simulink library "Control_System_Library"  (Simulink 8.0)
settings: Solver=ode45  StartTime=0.0  StopTime=10.0  RelTol=1e-3
values from neighbouring files (symbols this model uses):
  B_bias = [0 0 0]    [Initialize_UKF_Function.m]
  B_Init_Inertial = wrldmagm(Alt, Lat, Long, 2013)*1E-9    [Initialize_UKF_Function.m]
  I_c = [3.4 3.4 1.9]    [Initialize_UKF_Function.m]    (also in UKF_quaternion_withBias.m)
  NED_Init = dcmecef2ned(Lat, Long)*ECEF_Init    [Initialize_UKF_Function.m]
  q_i_s0 = init_attitude    [Initialize_UKF_Function.m]
  q_s_c = [1 0 0 0]    [Initialize_UKF_Function.m]    (also in Satellite2Controller_Conversion.m = dcm2quat(R); UKF_quaternion_withBias.m = [1; 0; 0; 0])
  Time_Start = 0    [Initialize_UKF_Function.m]
  Ts = .1    (= 0.1)    [Initialize_UKF_Function.m]
  w_bias = 0*[0.5 0.2 0.15]    [Initialize_UKF_Function.m]    (also in UKF_quaternion_withBias.m = zeros(3,1))
  w_init_s = [rand_w_x rand_w_y rand_w_z]    [Initialize_UKF_Function.m]
undefined symbols (not defined in the file or in its folder): aeroassertmsg, c, cd, DiscIntNeverNeededParam, dyear, Earth, epoch, fm, fn, k, maxdef, Newton, Raphson, sgp4, snorm, WGS84
libraries: commnoisgen2 x6, aerolibconvert2 x4, simulink x3, aerolibutil x2, aerolibtransform2 x2, dspmtrx3 x1, aerolibgravitysys x1
(part 3 of 3)

== matlab function Dynamic Model/Aerodynamic and Atmospheric Disturbance Torque Model/MATLAB Function1 ==
  data: Solar_Torque output double
function Solar_Torque = Solar_Drag_Torque()
% Solar_Drag_Torque
% Author: Brandon Jackson
% Contact: bajackso@mtu.edu
% Date: 26 June 2013
%
% Description: This function performs an analysis on the solar density
% above a fixed location of the Earth for the course of 1 day and 4 years
% to demonstrate that the atmospheric drag remains relatively constant
% during a given time period. This function does not account for f107
% models.

% Constant Definition
Fs = 1367;                  % Solar constant (W/m^2)
c = 3E8;                    % Speed of light (m/s)
r_cg = [0.2054; 0.2100; 0.2984];  % Center of gravity
r_cp = [0.2075; 0.2075; 0.3714];  % Center or pressure
r_cpcg = r_cp - r_cg;           % Radius from CG to CP (m)
A = [0.309; 0.309; 0.658];        % Surface area (m^2)
q = 0.75;

Solar_Torque = (Fs*A/c)*(1+q).*r_cpcg;

== matlab function Dynamic Model/Gravity Gradient Disturbance Torque Model/MATLAB Function ==
  data: R input double; G_grav output double
function G_grav = Gravity_Gradient_Torque(R)
% % G_grav = [0; 0; 0];
% 
% % Gravity_Gradient_Torque
% % Author: Brandon Jackson
% % Contact: bajackso@mtu.edu
% % Date: 3 June 2013
% %
%
% Constant Definitions
muC = 398600.4418*(1000^3);  % Earth gravitational parameter (km^3/s^2)
R_avg_earth = 6731*1000;     % (m)
Ixx = 4.3;
Iyy = 4.3;
Izz = 1.9;

R_sat = (R_avg_earth + R);

% Calculate the gravity gradient torques
G_grav = 3*muC/sum(R_sat.^5)*[(Izz-Iyy)*R_sat(2)*R_sat(3);...
    (Izz - Ixx)*R_sat(3)*R_sat(1); (Iyy-Ixx)*R_sat(1)*R_sat(3)];

== matlab function Dynamic Model/Kinematic Equations/MATLAB Function1 ==
  data: B output double; EA input double; Q output double
function [B,Q] = EulerAngle2Quat(EA)
%#codegen

% Prealocate
B = zeros(3,3);
Q = zeros(4,1);

% coder.extrinsic('dcm2quat');
DCM = [cos(EA(2,1))*cos(EA(1,1)) cos(EA(2,1))*sin(EA(1,1)) -sin(EA(2,1));
sin(EA(3,1))*sin(EA(2,1))*cos(EA(1,1))-cos(EA(3,1))*sin(EA(1,1)) sin(EA(3,1))*sin(EA(2,1))*sin(EA(1,1))+cos(EA(3,1))*cos(EA(1,1)) sin(EA(3,1))*cos(EA(2,1));
cos(EA(3,1))*sin(EA(2,1))*cos(EA(1,1))+sin(EA(3,1))*sin(EA(1,1)) cos(EA(3,1))*sin(EA(2,1))*sin(EA(1,1))-sin(EA(3,1))*cos(EA(1,1)) cos(EA(3,1))*cos(EA(2,1))];

Q = dcm2quat_c(DCM)';

B = 1/cos(EA(2,1))*[0 sin(EA(3,1)) cos(EA(3,1)); 
    0 cos(EA(2,1))*cos(EA(3,1)) -cos(EA(2,1))*sin(EA(3,1)); 
    cos(EA(2,1)) sin(EA(2,1))*sin(EA(3,1)) sin(EA(2,1))*cos(EA(3,1))];

end

function q = dcm2quat_c( dcm )
%  DCM2QUAT Convert direction cosine matrix to quaternion.
%   Q = DCM2QUAT( N ) calculates the quaternion, Q, for given
%   direction cosine matrix, N.   Input N is a 3-by-3-by-M matrix of
%   orthogonal direction cosine matrices.  The direction cosine matrix performs the
%   coordinate transformation of a vector in inertial axes to a vector in
%   body axes.  Q returns an M-by-4 matrix containing M quaternions. Q has
%   its scalar number as the first column.
%
%   Examples:
%
%   Determine the quaternion from direction cosine matrix:
%      dcm = [0 1 0; 1 0 0; 0 0 1];
%      q = dcm2quat(dcm)
%
%   Determine the quaternions from multiple direction cosine matrices:
%      dcm        = [ 0 1 0; 1 0 0; 0 0 1];
%      dcm(:,:,2) = [ 0.4330    0.2500   -0.8660; ...
%                     0.1768    0.9186    0.3536; ...
%                     0.8839   -0.3062    0.3536];
%      q = dcm2quat(dcm)
%
%   See also ANGLE2DCM, DCM2ANGLE, QUAT2DCM, QUAT2ANGLE, ANGLE2QUAT.

%   Copyright 2000-2010 The MathWorks, Inc.
%   $Revision: 1.1.6.5 $  $Date: 2010/09/28 03:13:59 $

q = zeros(1,4);
if any(~isreal(dcm) || ~isnumeric(dcm))
    error(message('aero:dcm2quat:isNotReal'));
end

if ((size(dcm,1) ~= 3) || (size(dcm,2) ~= 3))
    error(message('aero:dcm2quat:wrongDimension'));
end

tr = trace(dcm(:,:));

if (tr > 0)
    sqtrp1 = sqrt( tr + 1.0 );
    
    q(1,1) = 0.5*sqtrp1;
    q(1,2) = (dcm(2, 3) - dcm(3, 2))/(2.0*sqtrp1);
    q(1,3) = (dcm(3, 1) - dcm(1, 3))/(2.0*sqtrp1);
    q(1,4) = (dcm(1, 2) - dcm(2, 1))/(2.0*sqtrp1);
else
    d = diag(dcm(:,:));
    if ((d(2) > d(1)) && (d(2) > d(3)))
        % max value at dcm(2,2,i)
        sqdip1 = sqrt(d(2) - d(1) - d(3) + 1.0 );
        
        q(1,3) = 0.5*sqdip1;
        
        if ( sqdip1 ~= 0 )
            sqdip1 = 0.5/sqdip1;
        end
        
        q(1,1) = (dcm(3, 1) - dcm(1, 3))*sqdip1;
        q(1,2) = (dcm(1, 2) + dcm(2, 1))*sqdip1;
        q(1,4) = (dcm(2, 3) + dcm(3, 2))*sqdip1;
    elseif (d(3) > d(1))
        % max value at dcm(3,3,i)
        sqdip1 = sqrt(d(3) - d(1) - d(2) + 1.0 );
        
        q(1,4) = 0.5*sqdip1;
        
        if ( sqdip1 ~= 0 )
            sqdip1 = 0.5/sqdip1;
        end
        
        q(1,1) = (dcm(1, 2) - dcm(2, 1))*sqdip1;
        q(1,2) = (dcm(3, 1) + dcm(1, 3))*sqdip1;
        q(1,3) = (dcm(2, 3) + dcm(3, 2))*sqdip1;
    else
        % max value at dcm(1,1,i)
        sqdip1 = sqrt(d(1) - d(2) - d(3) + 1.0 );
        
        q(1,2) = 0.5*sqdip1;
        
        if ( sqdip1 ~= 0 )
            sqdip1 = 0.5/sqdip1;
        end
        
        q(1,1) = (dcm(2, 3) - dcm(3, 2))*sqdip1;
        q(1,3) = (dcm(1, 2) + dcm(2, 1))*sqdip1;
        q(1,4) = (dcm(3, 1) + dcm(1, 3))*sqdip1;
    end
end
end

== matlab function Dynamic Model/Kinematic Equations/MATLAB Function2 ==
  data: I_c input double; w_init_s input double; Torque_s input double; q0_i_s input double; w_s output double; q_i_s output double; q_s_c input double; Ts input double
function [w_s, q_i_s]= Satellite_Kinematics(I_c, w_init_s, Torque_s, q0_i_s, q_s_c, Ts)
%#codegen

persistent w_c_km1 q_i_c_km1

% Convert torque from satellite to controller frame
Torque_c_temp = quatmultiply(quatmultiply(quatinv(q_s_c), [0; Torque_s]), q_s_c);
Torque_c = Torque_c_temp(2:4,1);

if  isempty(w_c_km1) || isempty(q_i_c_km1)
    % First time this function is run, pass through initial conditions
    w_s = w_init_s;
    q_i_s = q0_i_s;
    
    % Store for next time
    w_c_temp = quatmultiply(quatmultiply(quatinv(q_s_c), [0; w_s]), q_s_c);
    w_c_km1 = w_c_temp(2:4);
    q_i_c_km1 = quatmultiply(q_i_s, q_s_c);
else
    % Second time this function is run, time to integrate
    
    x_km1 = [q_i_c_km1; w_c_km1];
    
    for i=1:10;
    Ts_rk4=Ts/10;
    % Integrate
    k1 = Kinematics(x_km1, I_c, Torque_c);
    k2 = Kinematics(x_km1 + 0.5*k1*Ts_rk4, I_c, Torque_c);
    k3 = Kinematics(x_km1 + 0.5*k2*Ts_rk4, I_c, Torque_c);
    k4 = Kinematics(x_km1 + k3*Ts_rk4, I_c, Torque_c);
    
    x_k = x_km1 + (k1 + 2*k2 + 2*k3 + k4)*Ts_rk4/6;
    
    end
    
    % Store for next time
    q_i_c_km1 = x_k(1:4);
    w_c_km1 = x_k(5:7);
    
    % Rotate and return
    q_i_s = quatmultiply(q_i_c_km1, quatinv(q_s_c));
    w_s_temp = quatmultiply(quatmultiply(q_s_c, [0; w_c_km1]), quatinv(q_s_c));
    w_s = w_s_temp(2:4);
end

end

function output = skew_matrix(x)
% Returns the skew symmetric matrix of the input vector

output = [0 -x(3) x(2);...
    x(3) 0 -x(1);...
    -x(2) x(1) 0];
end

function results = Kinematics(x, I, Torque_c)
q = x(1:4);
w = x(5:7);
I = diag(I);

q_dot = 0.5.*[0 -w'; w -skew_matrix(w)]*q;
w_dot = I^(-1)*(-skew_matrix(w)*(I*w) + Torque_c);
% w_dot = [0; 0; 0];
% w_dot(1,1) = ( Torque_c(1) - w(2)*w(3)*(I(3,3) - I(2,2)) )/I(1,1);
% w_dot(2,1) = ( Torque_c(2) - w(1)*w(3)*(I(1,1) - I(3,3)) )/I(2,2);
% w_dot(3,1) = ( Torque_c(3) - w(1)*w(2)*(I(2,2) - I(1,1)) )/I(3,3);

results = [q_dot; w_dot];
end

function qres = quatmultiply(q, r)
q = q';
r = r';
% Calculate vector portion of quaternion product
% vec = s1*v2 + s2*v1 + cross(v1,v2)
vec = [q(:,1).*r(:,2) q(:,1).*r(:,3) q(:,1).*r(:,4)] + ...
         [r(:,1).*q(:,2) r(:,1).*q(:,3) r(:,1).*q(:,4)]+...
         [ q(:,3).*r(:,4)-q(:,4).*r(:,3) ...
           q(:,4).*r(:,2)-q(:,2).*r(:,4) ...
           q(:,2).*r(:,3)-q(:,3).*r(:,2)];

% Calculate scalar portion of quaternion product
% scalar = s1*s2 - dot(v1,v2)
scalar = q(:,1).*r(:,1) - q(:,2).*r(:,2) - ...
             q(:,3).*r(:,3) - q(:,4).*r(:,4);
    
qres = [scalar  vec]';
end

function qinv = quatinv(qin)

q_conj = [qin(1); -qin(2:4)];
qinv = q_conj./sqrt(sum(qin.^2));

end
